simulink model "Test_Logic_Operation_Bitwise_Shift"  (Simulink 8.7)
settings: Solver=VariableStepDiscrete  StartTime=0.0  StopTime=len  RelTol=1e-3
libraries: Logic_Operations_Lib x1
settings Model: Creator=uzivatel  LastModifiedBy=Jozko Mrkvicka
settings DebuggingCC: SolverPrmCheckMsg=warning  StateNameClashWarn=warning

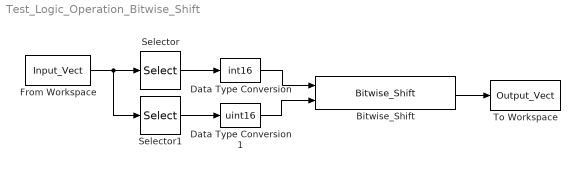
== system Test_Logic_Operation_Bitwise_Shift ==
  Bitwise_Shift : Logic_Operations_Lib/Logic_Operations_Lib/Bitwise_Shift
  Data Type Conversion : DataTypeConversion  OutDataTypeStr=int16
  Data Type Conversion1 : DataTypeConversion  OutDataTypeStr=uint16
  From Workspace : FromWorkspace  VariableName=Input_Vect  SampleTime=1  Interpolate=off  OutputAfterFinalValue=Holding final value
  Selector : Selector  IndexMode=Zero-based  InputPortWidth=2  SampleTime=1  IndexOptions=Index vector (dialog)  Indices=0  OutputSizes=1
  Selector1 : Selector  IndexMode=Zero-based  InputPortWidth=2  SampleTime=1  IndexOptions=Index vector (dialog)  Indices=1  OutputSizes=1
  To Workspace : ToWorkspace  VariableName=Output_Vect  SampleTime=1
  wires:
  Data Type Conversion1/1 -> Bitwise_Shift/2
  Data Type Conversion/1 -> Bitwise_Shift/1
  From Workspace/1 -> Selector1/1, Selector/1
  Bitwise_Shift/1 -> To Workspace/1
  Selector/1 -> Data Type Conversion/1
  Selector1/1 -> Data Type Conversion1/1
